simulink model "StraightACC_cs_old"  (R2016a)
settings: Solver=ode5  SolverMode=SingleTasking  StartTime=0.0  StopTime=10  FixedStep=1/1000  RelTol=1e-3
PreLoadFcn:
  | mbxruntime.callbacks.PreLoadFcn(bdroot);
PostLoadFcn:
  | mbxruntime.callbacks.PostLoadFcn(bdroot);
InitFcn:
  | mbxruntime.callbacks.InitFcn(bdroot);
StartFcn:
  | mbxruntime.callbacks.StartFcn(bdroot);
StopFcn:
  | mbxruntime.callbacks.StopFcn(bdroot);
model workspace (MAT data in the model file):
  mbox_table : struct (value not decoded)
  model_closed = 0
  sim_status = 0
values from neighbouring files (symbols this model uses):
  CCCDuration = 5    [PreScan_Runscript.m]
  V0 = CCCArray(2*CCCCasei-1)    [PreScan_Runscript.m]
  V1 = CCCArray(2*CCCCasei)    [PreScan_Runscript.m]
  VAccuracyIn = 0.8    [PreScan_Runscript.m]
  VDurationIn = 2    [PreScan_Runscript.m]
  VPIDIn = CCCArray(2*CCCCasei-1)    [PreScan_Runscript.m]
  VToleranceIn = 1    [PreScan_Runscript.m]
undefined symbols (not defined in the file or in its folder): ADASID, BMotor1, BMotor2, BrkDelayTime, DControlB, Delay1, Delay2, DiscIntNeverNeededParam, IControlB, JMotor1, JMotor2, PControlB, PreScanCarSimLoadFcn, ratioGearF, ratioGearR, TorqDelayTime, Tstep
undefined symbols (not defined in the file): WheelL0, WheelL1, WheelR0, WheelR1
libraries: simulink x13, simulink_extras x11, PreScanSimulinkLibrary x9, MyLib x3, Solver_SF x2, pil_lib x1, PreScanUsefulBlocks x1
(part 2 of 9)

== system StraightACC_cs_old/WheelL1_Roewe_550_S_Sedan_1 ==
  WheelL1_Roewe_550_S_Sedan_1 : Inport  Tag=inport/JointActuator  OutDataTypeStr=Bus: PRESCAN_POSE_DATA  SampleTime=10/1000  BusOutputAsStruct=on
  Actuator : Subsystem  Tag=VisuJoint  mask(PreScan Sink Block: VisuJoint){UniqueID=29, Translate_ObjectID3D=Roewe_550_S_Sedan_1.WheelL1, Rotate_ObjectID3D=Roewe_550_S_Sedan_1.WheelL1, TimeStep=10/1000, DisplayName=[]}
      mask prompts: UniqueID "Parent Unique ID"; Translate_ObjectID3D "Translate Object Name"; Rotate_ObjectID3D "Rotate Object Name"; TimeStep "Simulation Step"; DisplayName "Display Name"
      mask help:
      | The VisuJoint block provides a way to adapt the location and orientation of a part of an object.
      |
      | For more information, please click Help.
      settings: DeleteFcn=PreScanBlockDeleteFcn;
      mask Help: eval('openHelp(223)')
      mask Display: image(imread('Joint.png'))
  wires:
  WheelL1_Roewe_550_S_Sedan_1/1 -> Actuator/1(Joint)

== system StraightACC_cs_old/WheelR0_Roewe_550_S_Sedan_1 ==
  WheelR0_Roewe_550_S_Sedan_1 : Inport  Tag=inport/JointActuator  OutDataTypeStr=Bus: PRESCAN_POSE_DATA  SampleTime=10/1000  BusOutputAsStruct=on
  Actuator : Subsystem  Tag=VisuJoint  mask(PreScan Sink Block: VisuJoint){UniqueID=29, Translate_ObjectID3D=Roewe_550_S_Sedan_1.WheelR0, Rotate_ObjectID3D=Roewe_550_S_Sedan_1.WheelR0, TimeStep=10/1000, DisplayName=[]}
      mask prompts: UniqueID "Parent Unique ID"; Translate_ObjectID3D "Translate Object Name"; Rotate_ObjectID3D "Rotate Object Name"; TimeStep "Simulation Step"; DisplayName "Display Name"
      mask help:
      | The VisuJoint block provides a way to adapt the location and orientation of a part of an object.
      |
      | For more information, please click Help.
      settings: DeleteFcn=PreScanBlockDeleteFcn;
      mask Help: eval('openHelp(223)')
      mask Display: image(imread('Joint.png'))
  wires:
  WheelR0_Roewe_550_S_Sedan_1/1 -> Actuator/1(Joint)

== system StraightACC_cs_old/WheelR1_Roewe_550_S_Sedan_1 ==
  WheelR1_Roewe_550_S_Sedan_1 : Inport  Tag=inport/JointActuator  OutDataTypeStr=Bus: PRESCAN_POSE_DATA  SampleTime=10/1000  BusOutputAsStruct=on
  Actuator : Subsystem  Tag=VisuJoint  mask(PreScan Sink Block: VisuJoint){UniqueID=29, Translate_ObjectID3D=Roewe_550_S_Sedan_1.WheelR1, Rotate_ObjectID3D=Roewe_550_S_Sedan_1.WheelR1, TimeStep=10/1000, DisplayName=[]}
      mask prompts: UniqueID "Parent Unique ID"; Translate_ObjectID3D "Translate Object Name"; Rotate_ObjectID3D "Rotate Object Name"; TimeStep "Simulation Step"; DisplayName "Display Name"
      mask help:
      | The VisuJoint block provides a way to adapt the location and orientation of a part of an object.
      |
      | For more information, please click Help.
      settings: DeleteFcn=PreScanBlockDeleteFcn;
      mask Help: eval('openHelp(223)')
      mask Display: image(imread('Joint.png'))
  wires:
  WheelR1_Roewe_550_S_Sedan_1/1 -> Actuator/1(Joint)

== system StraightACC_cs_old/Audi_A8_Sedan_1/SELF_Demux ==
  SELF : Inport  OutDataTypeStr=Bus: PRESCAN_SELFSENSORDATA
  Bus Selector : BusSelector  OutputSignals=PositionX,PositionY,PositionZ,OrientationRoll,OrientationPitch,OrientationYaw,Velocity,Yaw_rate,Lat,Long,Alt
  Demux2 : Demux  Outputs=3
  Gain : Gain  Gain=180/pi
  Gain1 : Gain  Gain=180/pi
  Vector Concatenate1 : Concatenate  NumInputs=3
  compas converter : Subsystem
  x [m] : Outport
  y [m] : Outport  Port=2
  z [m] : Outport  Port=3
  rotx [deg] : Outport  Port=4
  roty [deg] : Outport  Port=5
  rotz [deg] : Outport  Port=6
  GPS lat [deg] : Outport  Port=7
  GPS long [deg] : Outport  Port=8
  GPS alt [m] : Outport  Port=9
  velocity [m/s] : Outport  Port=10
  heading [deg] : Outport  Port=11
  yaw rate [deg/s] : Outport  Port=12
  wires:
  Bus Selector/11 -> GPS alt [m]/1  "<Alt>"
  Bus Selector/10 -> GPS long [deg]/1  "<Long>"
  Bus Selector/9 -> GPS lat [deg]/1  "<Lat>"
  Bus Selector/8 -> Gain1/1  "<Yaw_rate>"
  Bus Selector/7 -> velocity [m/s]/1  "<Velocity>"
  Bus Selector/6 -> compas converter/1(rotz [rad]), Vector Concatenate1/3  "<OrientationYaw>"
  Bus Selector/5 -> Vector Concatenate1/2  "<OrientationPitch>"
  Bus Selector/4 -> Vector Concatenate1/1  "<OrientationRoll>"
  Vector Concatenate1/1 -> Gain/1
  Bus Selector/3 -> z [m]/1  "<PositionZ>"
  Bus Selector/2 -> y [m]/1  "<PositionY>"
  Bus Selector/1 -> x [m]/1  "<PositionX>"
  SELF/1 -> Bus Selector/1
  Gain/1 -> Demux2/1
  Demux2/1 -> rotx [deg]/1
  Demux2/2 -> roty [deg]/1
  Demux2/3 -> rotz [deg]/1
  compas converter/1(heading [deg]) -> heading [deg]/1
  Gain1/1 -> yaw rate [deg/s]/1

== system StraightACC_cs_old/Audi_A8_Sedan_1/STATE_Audi_A8_Sedan_1 ==
  State : Inport  SampleTime=TimeStep
  Bus Creator : BusCreator  Inputs=15  OutDataTypeStr=Bus: PRESCAN_STATEACTUATORDATA  NonVirtualBus=on
  Demux : Demux  Outputs=15
  iniBODYAngles wrtVEH [rad] : Constant  Value=[Roll0 Pitch0 0]  SampleTime=TimeStep
  iniVEHAngles wrtGLOB [rad] : Constant  Value=[0 0 Yaw0]  SampleTime=TimeStep
  iniVEHposition wrtGLOB [m] : Constant  Value=[x0 y0 z0]  SampleTime=TimeStep
  state2FullState : PreScanSimulinkLibrary/state2FullState  SystemSampleTime=-1
  StateBus : Outport  OutDataTypeStr=Bus: PRESCAN_STATEACTUATORDATA
  wires:
  Bus Creator/1 -> StateBus/1
  State/1 -> state2FullState/1
  state2FullState/1 -> Demux/1
  iniVEHposition wrtGLOB [m]/1 -> state2FullState/2
  iniBODYAngles wrtVEH [rad]/1 -> state2FullState/3
  iniVEHAngles wrtGLOB [rad]/1 -> state2FullState/4
  Demux/1 -> Bus Creator/1  "PositionX"
  Demux/2 -> Bus Creator/2  "PositionY"
  Demux/3 -> Bus Creator/3  "PositionZ"
  Demux/4 -> Bus Creator/4  "VelocityX"
  Demux/5 -> Bus Creator/5  "VelocityY"
  Demux/6 -> Bus Creator/6  "VelocityZ"
  Demux/7 -> Bus Creator/7  "AccelerationX"
  Demux/8 -> Bus Creator/8  "AccelerationY"
  Demux/9 -> Bus Creator/9  "AccelerationZ"
  Demux/10 -> Bus Creator/10  "OrientationRoll"
  Demux/11 -> Bus Creator/11  "OrientationPitch"
  Demux/12 -> Bus Creator/12  "OrientationYaw"
  Demux/13 -> Bus Creator/13  "AngularVelocityRoll"
  Demux/14 -> Bus Creator/14  "AngularVelocityPitch"
  Demux/15 -> Bus Creator/15  "AngularVelocityYaw"

== system StraightACC_cs_old/Audi_A8_Sedan_1/Trajectories ==
  Traj2State1 : Subsystem  Tag=Traj2State  mask(PreScan Demux Block:){}
      settings: DeleteFcn=PreScanBlockDeleteFcn;
  TrajCoGOffset : Subsystem  Tag=TrajCoGOffset  mask(Trajectory CoG Offset block){CoGOffsetZ=0.55, InitRoll=0, InitPitch=0}
      mask prompts: CoGOffsetZ "Z-component of CoG Offset [m]:"; InitRoll "Initial Roll angle [deg]:"; InitPitch "Initial Pitch angle [deg]:"
      mask help: A trajectory follows the surface of the road. However the position of a actor is based on the actor's Center of Gravity, which is typically above the road. This block converts from the trajectory along the road surface to the trajectory of the actor's CoG by realigning the z-component of the CoG offset to be normal to the road.
      settings: DeleteFcn=PreScanBlockDeleteFcn;
  Trajectory_1 : Subsystem  Tag=Trajectory  mask(PreScan Source Block: Trajectory){FileName='Trajectory_1.mat', TimeStep=10/1000}
      mask prompts: TimeStep "Time Step [s]"
      mask help:
      | The Trajectory block contains the trajectories defined in the PreScan Experiment Editor. The output of the trajectory block is the (vehicle) State.
      |
      | For more information, please click Help.
      mask init:
      | EXPROOT=pwd;  % TODO better construction for locating base experiment
      | 
      | trajfilename = fullfile(EXPROOT,'Trajectories',FileName);
      | load(trajfilename);
      | trajectory=trajectory';
      | 
      | traj.time=trajectory(:,1);%[];
      | traj.signals.values=trajectory(:,2:19);
      | traj.dimensions=18;
      | traj.label='';
      | 
      | SampleTime=traj.time(2)-traj.time(1);
      settings: DeleteFcn=PreScanBlockDeleteFcn;
      mask Help: eval('openHelp(312)')
      mask Display: fprintf(FileName)
  Trajectory_1_Offset : Constant  Tag=TrajectoryOffset  Value="[0  0  0  0  0  0]"
  State : Outport  Tag=TrajOutport
  wires:
  Trajectory_1/1(trajectory) -> Traj2State1/1(Traj Org)
  Trajectory_1_Offset/1 -> Traj2State1/2(Offset)
  TrajCoGOffset/1(State Out) -> State/1
  Traj2State1/1(state) -> TrajCoGOffset/1(State In)

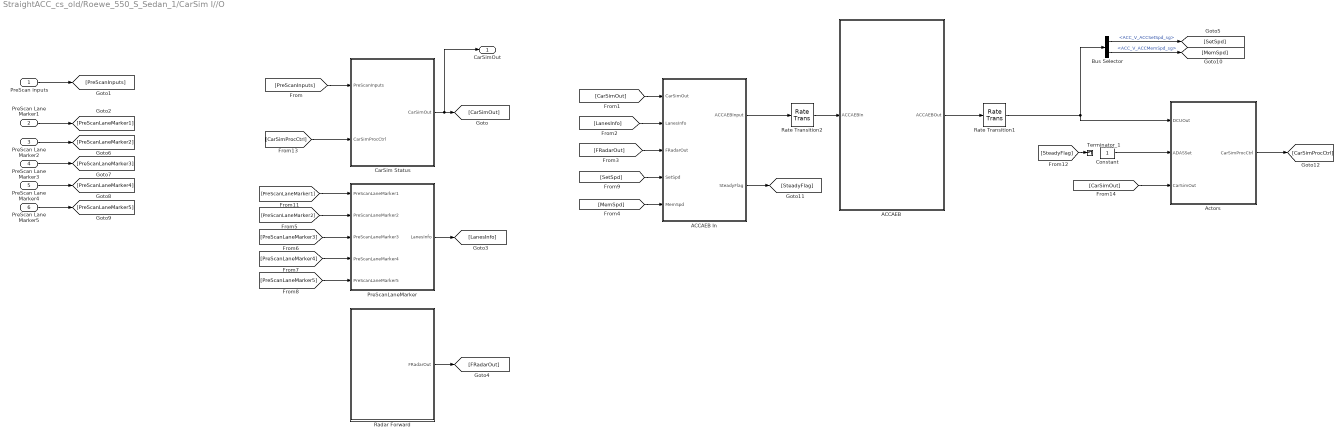
== system StraightACC_cs_old/Roewe_550_S_Sedan_1/CarSim I//O ==
  PreScan inputs : Inport
  PreScan Lane Marker1 : Inport  Port=2
  PreScan Lane Marker2 : Inport  Port=3
  PreScan Lane Marker3 : Inport  Port=4
  PreScan Lane Marker4 : Inport  Port=5
  PreScan Lane Marker5 : Inport  Port=6
  ACCAEB : Subsystem  DialogController=pil_create_dialog  LoadFcn=|
      | try
      |    if ~strcmp(rtw.pil.getPILVersion, '6.10 (R2016a)_12')
      |       set_param(gcb, 'DialogController', '');
      |       set_param(gcb, 'DialogControllerArgs', '');
      |    end
      | catch e
      |       set_param(gcb, 'DialogController', '');
      |       set_param(gcb, 'DialogControllerArgs', '');
      | end
      mask help: PIL:pil:XILBlockMaskDesc
      mask Display: disp('SIL S-Function');
  ACCAEB In : Subsystem  TreatAsAtomicUnit=on
  Actors : Subsystem
  Bus Selector : BusSelector  OutputSignals=ACC_V_ACCSetSpd_sg,ACC_V_ACCMemSpd_sg
  "CarSim Status " : Subsystem  TreatAsAtomicUnit=on
  Constant : Constant
  PreScanLaneMarker : Subsystem  TreatAsAtomicUnit=on
  Radar Forward : Subsystem  TreatAsAtomicUnit=on
  Rate Transition1 : RateTransition  OutPortSampleTime=0.001
  Rate Transition2 : RateTransition  OutPortSampleTime=0.01
  Terminator_1 : Terminator
  CarSimOut : Outport
  wires:
  [PreScanInputs] -> "CarSim Status "/1(PreScanInputs)
  PreScan inputs/1 -> [PreScanInputs]
  PreScan Lane Marker1/1 -> [PreScanLaneMarker1]
  "CarSim Status "/1(CarSimOut) -> CarSimOut/1, [CarSimOut]
  [PreScanLaneMarker1] -> PreScanLaneMarker/1(PreScanLaneMarker1)
  [CarSimOut] -> ACCAEB In/1(CarSimOut)
  PreScanLaneMarker/1(LanesInfo) -> [LanesInfo]
  [LanesInfo] -> ACCAEB In/2(LanesInfo)
  Radar Forward/1(FRadarOut) -> [FRadarOut]
  [FRadarOut] -> ACCAEB In/3(FRadarOut)
  [CarSimProcCtrl] -> "CarSim Status "/2(CarSimProcCtrl)
  PreScan Lane Marker2/1 -> [PreScanLaneMarker2]
  PreScan Lane Marker3/1 -> [PreScanLaneMarker3]
  PreScan Lane Marker4/1 -> [PreScanLaneMarker4]
  PreScan Lane Marker5/1 -> [PreScanLaneMarker5]
  [PreScanLaneMarker2] -> PreScanLaneMarker/2(PreScanLaneMarker2)
  [PreScanLaneMarker3] -> PreScanLaneMarker/3(PreScanLaneMarker3)
  [PreScanLaneMarker4] -> PreScanLaneMarker/4(PreScanLaneMarker4)
  [PreScanLaneMarker5] -> PreScanLaneMarker/5(PreScanLaneMarker5)
  Rate Transition2/1 -> ACCAEB/1(ACCAEBIn)
  ACCAEB In/1(ACCAEBInput) -> Rate Transition2/1
  ACCAEB/1(ACCAEBOut) -> Rate Transition1/1
  Rate Transition1/1 -> Bus Selector/1, Actors/1(DCUOut)
  ACCAEB In/2(SteadyFlag) -> [SteadyFlag]
  [CarSimOut] -> Actors/3(CarSimOut)
  Actors/1(CarSimProcCtrl) -> [CarSimProcCtrl]
  Constant/1 -> Actors/2(ADASSet)
  Bus Selector/1 -> [SetSpd]  "<ACC_V_ACCSetSpd_sg>"
  Bus Selector/2 -> [MemSpd]  "<ACC_V_ACCMemSpd_sg>"
  [SetSpd] -> ACCAEB In/4(SetSpd)
  [MemSpd] -> ACCAEB In/5(MemSpd)
  [SteadyFlag] -> Terminator_1/1

== system StraightACC_cs_old/Roewe_550_S_Sedan_1/CarSim_Vehicle ==
  note: For state mode 'Dynamic' positions
      | are not taken into account, as they
      | are computed by integrating velocity.
      | Click annotation for Help.
  Contact_In : Inport
  CarSim S-Function2 : Solver_SF/CarSim S-Function2  Priority=1  VehicleCode=i_i  SIMFILE=simfile.sim
      settings: AttributesFormatString=Vehicle Code: %<VehicleCode>
  CarSim2PreScanSTATE : Subsystem  Tag=CarSim2PreScanSTATE  mask(CarSim2PreScan:){z0=0}
      mask prompts: z0 "PreScan Actor initial COG z-position wrt GLOBAL axis system [m]"
      mask help: This block converts the outputs coming from the CarSim block into consistent PreScan signals.
  CarSim2PreScan_BUS : Subsystem  Tag=CarSim2PreScan_BUS  mask(PreScan block: CarSim to PreScan BUS){TyreRadius=0.44999998807907104, cogZOffset=0}
      mask prompts: TyreRadius "Tyre Radius [m]"; cogZOffset "cog Z offset [m]"
      mask help: CarSim to PreScan BUS selector
      mask Help: eval('openHelp()')
      mask Display: disp('PreScan BUS\nVehicleDynamics')
  CarSim2PreScan_ContactAdapter : Subsystem  Tag=CarSim2PreScan_ContactAdapter  mask{wheelRadius=0.44999998807907104}
      mask prompts: wheelRadius "Wheel radius:"
  MuxState : Subsystem  Tag=mux/State  mask(Empty Dynamics State Block){positioningmode=on, TimeStep=1/1000}
      mask prompts: positioningmode "Positioning Mode"; TimeStep "Auto Assigned: Time Step [s]"
      mask help:
      | Build the state of an actor based on user input.
      | The user can either use positioning mode or dynamics mode.
      | - When using positioning mode the position and orientation of the actor are set directly based on the input. Expected input is relative to the initial position and orientation of the actor. It's also possible to specify the velocity of the actor, though this input isn't used, only passed on.
      | - When using dynamics mode the position input is ignored. Expected input is velocity and orientation. The velocity is relative the current orientation of the actor, while orientation is relative to its initial orientation. The position of the actor is calculated based on the velocity and orientation given.
      settings: DeleteFcn=PreScanBlockDeleteFcn;
  TyreContact To Road Information : Subsystem  Tag=TyreContactToRoadInformation  mask{Roll0=0, Pitch0=0, Yaw0=0}
      mask prompts: Roll0 "Ini roll-angle BODY wrt VEHICLE axis system [deg]"; Pitch0 "Ini pitch-angle BODY wrt VEHICLE axis system [deg]"; Yaw0 "Ini yaw-angle VEHICLE wrt GLOBAL axis system [deg]"
  State : Outport
  State_BUS : Outport  Port=2
  ContactParams : Outport  Port=3
  wires:
  MuxState/1(state) -> State/1, CarSim2PreScan_ContactAdapter/1(State)
  CarSim2PreScanSTATE/1(x [m]) -> MuxState/1(x [m])
  CarSim2PreScanSTATE/2(y [m]) -> MuxState/2(y [m])
  CarSim2PreScanSTATE/3(z [m]) -> MuxState/3(z [m])
  CarSim2PreScanSTATE/4(dx [m/s]) -> MuxState/4(dx [m/s])
  CarSim2PreScanSTATE/5(dy [m/s]) -> MuxState/5(dy [m/s])
  CarSim2PreScanSTATE/6(dz [m/s]) -> MuxState/6(dz [m/s])
  CarSim2PreScanSTATE/7(R [rad]) -> MuxState/7(R [rad])
  CarSim2PreScanSTATE/8(P [rad]) -> MuxState/8(P [rad])
  CarSim2PreScanSTATE/9(Y [rad]) -> MuxState/9(Y [rad])
  CarSim2PreScan_BUS/1(PreScanBUS_VehicleDynamics) -> State_BUS/1, CarSim2PreScan_ContactAdapter/2(State_Bus)
  CarSim S-Function2/1 -> CarSim2PreScanSTATE/1(CarSim_In), CarSim2PreScan_BUS/1(CarSim_In)
  Contact_In/1 -> TyreContact To Road Information/1(TyreInfo_in)
  CarSim2PreScan_ContactAdapter/1(ContactParams) -> ContactParams/1

== system StraightACC_cs_old/Roewe_550_S_Sedan_1/LaneMarkerSensor_1_Data ==
  In1 : Inport
  Bus Creator : BusCreator  Inputs='SliceCount','ScanAtSensor','ScanAtDistance1','ScanAtDistance2','ScanAtDistance3'
  Constant : Constant
  Constant1 : Constant  Value=NUMBEROFSLICES
  Constant2 : Constant  Value=2
  Constant3 : Constant  Value=3
  Constant4 : Constant  Value=4
  Data Type Conversion : DataTypeConversion  OutDataTypeStr=int32
  If{,1..3} (4 alike) : If  NumInputs=2  IfExpression=u1 >= u2  ShowElse=off
  If Action Subsystem1 : Subsystem  TreatAsAtomicUnit=on
  If Action Subsystem2 : Subsystem  TreatAsAtomicUnit=on
  If Action Subsystem3 : Subsystem  TreatAsAtomicUnit=on
  If Action Subsystem4 : Subsystem  TreatAsAtomicUnit=on
  Merge{,1..3} (4 alike) : Merge  InitialOutput=0
  Zero-filled data bus{,1..3} (4 alike) : Constant  Value=0  VectorParams1D=off  OutDataTypeStr=Bus: PRESCAN_LANEMARKER_DATA  SampleTime=TimeStep
  Detection Data : Outport
  wires:
  Data Type Conversion/1 -> Bus Creator/1  "SliceCount"
  In1/1 -> If Action Subsystem2/1(In1), If Action Subsystem4/1(In1), If Action Subsystem3/1(In1), If Action Subsystem1/1(In1)
  Zero-filled data bus3/1 -> Merge3/1
  Zero-filled data bus2/1 -> Merge2/1
  Zero-filled data bus1/1 -> Merge1/1
  Zero-filled data bus/1 -> Merge/1
  Merge3/1 -> Bus Creator/5  "ScanAtDistance3"
  Merge2/1 -> Bus Creator/4  "ScanAtDistance2"
  Merge1/1 -> Bus Creator/3  "ScanAtDistance1"
  If3/1 -> If Action Subsystem4/Action
  If Action Subsystem4/1(Out1) -> Merge3/2
  Constant4/1 -> If3/2, If Action Subsystem4/2(In2)
  If2/1 -> If Action Subsystem3/Action
  If Action Subsystem3/1(Out1) -> Merge2/2
  Constant3/1 -> If Action Subsystem3/2(In2), If2/2
  If1/1 -> If Action Subsystem1/Action
  If Action Subsystem1/1(Out1) -> Merge1/2
  Constant2/1 -> If Action Subsystem1/2(In2), If1/2
  Merge/1 -> Bus Creator/2  "ScanAtSensor"
  Bus Creator/1 -> Detection Data/1
  If/1 -> If Action Subsystem2/Action
  If Action Subsystem2/1(Out1) -> Merge/2
  Constant/1 -> If Action Subsystem2/2(In2), If/2
  Constant1/1 -> Data Type Conversion/1, If3/1, If2/1, If1/1, If/1

== system StraightACC_cs_old/Roewe_550_S_Sedan_1/LaneMarkerSensor_2_Data ==
  In1 : Inport
  Bus Creator : BusCreator  Inputs='SliceCount','ScanAtSensor','ScanAtDistance1','ScanAtDistance2','ScanAtDistance3'
  Constant : Constant
  Constant1 : Constant  Value=NUMBEROFSLICES
  Constant2 : Constant  Value=2
  Constant3 : Constant  Value=3
  Constant4 : Constant  Value=4
  Data Type Conversion : DataTypeConversion  OutDataTypeStr=int32
  If{,1..3} (4 alike) : If  NumInputs=2  IfExpression=u1 >= u2  ShowElse=off
  If Action Subsystem1 : Subsystem  TreatAsAtomicUnit=on
  If Action Subsystem2 : Subsystem  TreatAsAtomicUnit=on
  If Action Subsystem3 : Subsystem  TreatAsAtomicUnit=on
  If Action Subsystem4 : Subsystem  TreatAsAtomicUnit=on
  Merge{,1..3} (4 alike) : Merge  InitialOutput=0
  Zero-filled data bus{,1..3} (4 alike) : Constant  Value=0  VectorParams1D=off  OutDataTypeStr=Bus: PRESCAN_LANEMARKER_DATA  SampleTime=TimeStep
  Detection Data : Outport
  wires:
  Data Type Conversion/1 -> Bus Creator/1  "SliceCount"
  In1/1 -> If Action Subsystem2/1(In1), If Action Subsystem4/1(In1), If Action Subsystem3/1(In1), If Action Subsystem1/1(In1)
  Zero-filled data bus3/1 -> Merge3/1
  Zero-filled data bus2/1 -> Merge2/1
  Zero-filled data bus1/1 -> Merge1/1
  Zero-filled data bus/1 -> Merge/1
  Merge3/1 -> Bus Creator/5  "ScanAtDistance3"
  Merge2/1 -> Bus Creator/4  "ScanAtDistance2"
  Merge1/1 -> Bus Creator/3  "ScanAtDistance1"
  If3/1 -> If Action Subsystem4/Action
  If Action Subsystem4/1(Out1) -> Merge3/2
  Constant4/1 -> If3/2, If Action Subsystem4/2(In2)
  If2/1 -> If Action Subsystem3/Action
  If Action Subsystem3/1(Out1) -> Merge2/2
  Constant3/1 -> If Action Subsystem3/2(In2), If2/2
  If1/1 -> If Action Subsystem1/Action
  If Action Subsystem1/1(Out1) -> Merge1/2
  Constant2/1 -> If Action Subsystem1/2(In2), If1/2
  Merge/1 -> Bus Creator/2  "ScanAtSensor"
  Bus Creator/1 -> Detection Data/1
  If/1 -> If Action Subsystem2/Action
  If Action Subsystem2/1(Out1) -> Merge/2
  Constant/1 -> If Action Subsystem2/2(In2), If/2
  Constant1/1 -> Data Type Conversion/1, If3/1, If2/1, If1/1, If/1

== system StraightACC_cs_old/Roewe_550_S_Sedan_1/LaneMarkerSensor_3_Data ==
  In1 : Inport
  Bus Creator : BusCreator  Inputs='SliceCount','ScanAtSensor','ScanAtDistance1','ScanAtDistance2','ScanAtDistance3'
  Constant : Constant
  Constant1 : Constant  Value=NUMBEROFSLICES
  Constant2 : Constant  Value=2
  Constant3 : Constant  Value=3
  Constant4 : Constant  Value=4
  Data Type Conversion : DataTypeConversion  OutDataTypeStr=int32
  If{,1..3} (4 alike) : If  NumInputs=2  IfExpression=u1 >= u2  ShowElse=off
  If Action Subsystem1 : Subsystem  TreatAsAtomicUnit=on
  If Action Subsystem2 : Subsystem  TreatAsAtomicUnit=on
  If Action Subsystem3 : Subsystem  TreatAsAtomicUnit=on
  If Action Subsystem4 : Subsystem  TreatAsAtomicUnit=on
  Merge{,1..3} (4 alike) : Merge  InitialOutput=0
  Zero-filled data bus{,1..3} (4 alike) : Constant  Value=0  VectorParams1D=off  OutDataTypeStr=Bus: PRESCAN_LANEMARKER_DATA  SampleTime=TimeStep
  Detection Data : Outport
  wires:
  Data Type Conversion/1 -> Bus Creator/1  "SliceCount"
  In1/1 -> If Action Subsystem2/1(In1), If Action Subsystem4/1(In1), If Action Subsystem3/1(In1), If Action Subsystem1/1(In1)
  Zero-filled data bus3/1 -> Merge3/1
  Zero-filled data bus2/1 -> Merge2/1
  Zero-filled data bus1/1 -> Merge1/1
  Zero-filled data bus/1 -> Merge/1
  Merge3/1 -> Bus Creator/5  "ScanAtDistance3"
  Merge2/1 -> Bus Creator/4  "ScanAtDistance2"
  Merge1/1 -> Bus Creator/3  "ScanAtDistance1"
  If3/1 -> If Action Subsystem4/Action
  If Action Subsystem4/1(Out1) -> Merge3/2
  Constant4/1 -> If3/2, If Action Subsystem4/2(In2)
  If2/1 -> If Action Subsystem3/Action
  If Action Subsystem3/1(Out1) -> Merge2/2
  Constant3/1 -> If Action Subsystem3/2(In2), If2/2
  If1/1 -> If Action Subsystem1/Action
  If Action Subsystem1/1(Out1) -> Merge1/2
  Constant2/1 -> If Action Subsystem1/2(In2), If1/2
  Merge/1 -> Bus Creator/2  "ScanAtSensor"
  Bus Creator/1 -> Detection Data/1
  If/1 -> If Action Subsystem2/Action
  If Action Subsystem2/1(Out1) -> Merge/2
  Constant/1 -> If Action Subsystem2/2(In2), If/2
  Constant1/1 -> Data Type Conversion/1, If3/1, If2/1, If1/1, If/1

== system StraightACC_cs_old/Roewe_550_S_Sedan_1/LaneMarkerSensor_4_Data ==
  In1 : Inport
  Bus Creator : BusCreator  Inputs='SliceCount','ScanAtSensor','ScanAtDistance1','ScanAtDistance2','ScanAtDistance3'
  Constant : Constant
  Constant1 : Constant  Value=NUMBEROFSLICES
  Constant2 : Constant  Value=2
  Constant3 : Constant  Value=3
  Constant4 : Constant  Value=4
  Data Type Conversion : DataTypeConversion  OutDataTypeStr=int32
  If{,1..3} (4 alike) : If  NumInputs=2  IfExpression=u1 >= u2  ShowElse=off
  If Action Subsystem1 : Subsystem  TreatAsAtomicUnit=on
  If Action Subsystem2 : Subsystem  TreatAsAtomicUnit=on
  If Action Subsystem3 : Subsystem  TreatAsAtomicUnit=on
  If Action Subsystem4 : Subsystem  TreatAsAtomicUnit=on
  Merge{,1..3} (4 alike) : Merge  InitialOutput=0
  Zero-filled data bus{,1..3} (4 alike) : Constant  Value=0  VectorParams1D=off  OutDataTypeStr=Bus: PRESCAN_LANEMARKER_DATA  SampleTime=TimeStep
  Detection Data : Outport
  wires:
  Data Type Conversion/1 -> Bus Creator/1  "SliceCount"
  In1/1 -> If Action Subsystem2/1(In1), If Action Subsystem4/1(In1), If Action Subsystem3/1(In1), If Action Subsystem1/1(In1)
  Zero-filled data bus3/1 -> Merge3/1
  Zero-filled data bus2/1 -> Merge2/1
  Zero-filled data bus1/1 -> Merge1/1
  Zero-filled data bus/1 -> Merge/1
  Merge3/1 -> Bus Creator/5  "ScanAtDistance3"
  Merge2/1 -> Bus Creator/4  "ScanAtDistance2"
  Merge1/1 -> Bus Creator/3  "ScanAtDistance1"
  If3/1 -> If Action Subsystem4/Action
  If Action Subsystem4/1(Out1) -> Merge3/2
  Constant4/1 -> If3/2, If Action Subsystem4/2(In2)
  If2/1 -> If Action Subsystem3/Action
  If Action Subsystem3/1(Out1) -> Merge2/2
  Constant3/1 -> If Action Subsystem3/2(In2), If2/2
  If1/1 -> If Action Subsystem1/Action
  If Action Subsystem1/1(Out1) -> Merge1/2
  Constant2/1 -> If Action Subsystem1/2(In2), If1/2
  Merge/1 -> Bus Creator/2  "ScanAtSensor"
  Bus Creator/1 -> Detection Data/1
  If/1 -> If Action Subsystem2/Action
  If Action Subsystem2/1(Out1) -> Merge/2
  Constant/1 -> If Action Subsystem2/2(In2), If/2
  Constant1/1 -> Data Type Conversion/1, If3/1, If2/1, If1/1, If/1

== system StraightACC_cs_old/Roewe_550_S_Sedan_1/LaneMarkerSensor_5_Data ==
  In1 : Inport
  Bus Creator : BusCreator  Inputs='SliceCount','ScanAtSensor','ScanAtDistance1','ScanAtDistance2','ScanAtDistance3'
  Constant : Constant
  Constant1 : Constant  Value=NUMBEROFSLICES
  Constant2 : Constant  Value=2
  Constant3 : Constant  Value=3
  Constant4 : Constant  Value=4
  Data Type Conversion : DataTypeConversion  OutDataTypeStr=int32
  If{,1..3} (4 alike) : If  NumInputs=2  IfExpression=u1 >= u2  ShowElse=off
  If Action Subsystem1 : Subsystem  TreatAsAtomicUnit=on
  If Action Subsystem2 : Subsystem  TreatAsAtomicUnit=on
  If Action Subsystem3 : Subsystem  TreatAsAtomicUnit=on
  If Action Subsystem4 : Subsystem  TreatAsAtomicUnit=on
  Merge{,1..3} (4 alike) : Merge  InitialOutput=0
  Zero-filled data bus{,1..3} (4 alike) : Constant  Value=0  VectorParams1D=off  OutDataTypeStr=Bus: PRESCAN_LANEMARKER_DATA  SampleTime=TimeStep
  Detection Data : Outport
  wires:
  Data Type Conversion/1 -> Bus Creator/1  "SliceCount"
  In1/1 -> If Action Subsystem2/1(In1), If Action Subsystem4/1(In1), If Action Subsystem3/1(In1), If Action Subsystem1/1(In1)
  Zero-filled data bus3/1 -> Merge3/1
  Zero-filled data bus2/1 -> Merge2/1
  Zero-filled data bus1/1 -> Merge1/1
  Zero-filled data bus/1 -> Merge/1
  Merge3/1 -> Bus Creator/5  "ScanAtDistance3"
  Merge2/1 -> Bus Creator/4  "ScanAtDistance2"
  Merge1/1 -> Bus Creator/3  "ScanAtDistance1"
  If3/1 -> If Action Subsystem4/Action
  If Action Subsystem4/1(Out1) -> Merge3/2
  Constant4/1 -> If3/2, If Action Subsystem4/2(In2)
  If2/1 -> If Action Subsystem3/Action
  If Action Subsystem3/1(Out1) -> Merge2/2
  Constant3/1 -> If Action Subsystem3/2(In2), If2/2
  If1/1 -> If Action Subsystem1/Action
  If Action Subsystem1/1(Out1) -> Merge1/2
  Constant2/1 -> If Action Subsystem1/2(In2), If1/2
  Merge/1 -> Bus Creator/2  "ScanAtSensor"
  Bus Creator/1 -> Detection Data/1
  If/1 -> If Action Subsystem2/Action
  If Action Subsystem2/1(Out1) -> Merge/2
  Constant/1 -> If Action Subsystem2/2(In2), If/2
  Constant1/1 -> Data Type Conversion/1, If3/1, If2/1, If1/1, If/1

== system StraightACC_cs_old/Roewe_550_S_Sedan_1/PreScan_RayCast_Contact_Sensor ==
  ContactParams : Inport  SampleTime=TimeStep
  Bus Creator2 : BusCreator  Inputs=4
  Constant : Constant  Value=0
  Contact Point Bus Creator : Subsystem
  Contact Point Bus Creator1 : Subsystem
  Contact Point Bus Creator2 : Subsystem
  Contact Point Bus Creator3 : Subsystem
  Demux : Demux
  Demux1 : Demux  Outputs=[9 1 12 4]
  Demux2 : Demux
  For All Wheel Contacts : Subsystem  TreatAsAtomicUnit=on
  Mux6 : Mux  Inputs=2
  Rate Transition : RateTransition  OutPortSampleTimeOpt=Inherit
  Subsystem1 : Subsystem  mask{NumberOfWheels=4, MaxContactPoints=1, Range=4}
      mask prompts: NumberOfWheels "Number of Wheels"; MaxContactPoints "Maximum number of Contact Points"
      mask Display: disp('RayCast Contact Sensor')
  Subsystem2 : Subsystem  mask{nrOfWheels=4}
      mask prompts: nrOfWheels "Number of Wheels:"
      mask Display:
      | port_label('input', 1,'Wheel poses')
      | port_label('input', 2,'Wheel radius')
      | port_label('input', 3,'Vehicle orientation')
      | 
      | port_label('output', 1,'Virtual poses')
  Vehicle Local to World : Subsystem
  Wheels = 4 : Subsystem  mask{NumberOfWheels=4}
      mask prompts: NumberOfWheels "Number of Wheels"
      mask Display:
      | port_label('input', 1,'Vehicle wrt World')
      | port_label('input', 2,'Wheels wrt World')
  Wheels Local to World : Subsystem  Tag=MuxWheels  mask(PreScan Mux Block:){}
      settings: DeleteFcn=PreScanBlockDeleteFcn;
  Results : Outport
  wires:
  Demux1/3 -> Demux2/1
  Demux1/1 -> Vehicle Local to World/1(State)
  ContactParams/1 -> Demux1/1
  Bus Creator2/1 -> Rate Transition/1
  Constant/1 -> Wheels Local to World/1(Steer Angle Front [deg]), Wheels Local to World/2(Steer Angle Rear [deg])
  Demux2/4 -> Wheels Local to World/7(Disp RR [m])
  Demux2/3 -> Wheels Local to World/6(Disp RL [m])
  Demux2/2 -> Wheels Local to World/5(Disp FR [m])
  Demux2/1 -> Wheels Local to World/4(Disp FL [m])
  Demux1/2 -> Wheels Local to World/3(Velocity [m/s])
  Wheels Local to World/1(Wheel Poses) -> Wheels = 4/2(Wheels wrt World)
  Vehicle Local to World/2(Orientation) -> Mux6/2, Subsystem2/3(Vehicle orientation)
  Vehicle Local to World/1(Position) -> Mux6/1
  Contact Point Bus Creator3/1(bus out) -> Bus Creator2/4  "TireRR"
  Contact Point Bus Creator2/1(bus out) -> Bus Creator2/3  "TireRL"
  Contact Point Bus Creator1/1(bus out) -> Bus Creator2/2  "TireFR"
  Contact Point Bus Creator/1(bus out) -> Bus Creator2/1  "TireFL"
  Demux/4 -> Contact Point Bus Creator3/1(demux in)
  Demux/3 -> Contact Point Bus Creator2/1(demux in)
  Demux/2 -> Contact Point Bus Creator1/1(demux in)
  Demux/1 -> Contact Point Bus Creator/1(demux in)
  Mux6/1 -> Wheels = 4/1(Vehicle wrt World)
  Rate Transition/1 -> Results/1
  Demux1/4 -> Subsystem2/2(Wheel radius)
  Wheels = 4/1(WheelPoses) -> Subsystem2/1(Wheel poses)
  Subsystem1/1(Out1) -> For All Wheel Contacts/1(In1)
  For All Wheel Contacts/1(Out1) -> Demux/1
  Subsystem2/1(Virtual Poses) -> Subsystem1/1(In1)

== system StraightACC_cs_old/Roewe_550_S_Sedan_1/PreScan_RayCast_Contact_Sensor1 ==
  ContactParams : Inport  SampleTime=TimeStep
  Bus Creator2 : BusCreator  Inputs=4
  Constant : Constant  Value=0
  Contact Point Bus Creator : Subsystem
  Contact Point Bus Creator1 : Subsystem
  Contact Point Bus Creator2 : Subsystem
  Contact Point Bus Creator3 : Subsystem
  Demux : Demux
  Demux1 : Demux  Outputs=[9 1 12 4]
  Demux2 : Demux
  For All Wheel Contacts : Subsystem  TreatAsAtomicUnit=on
  Mux6 : Mux  Inputs=2
  Rate Transition : RateTransition  OutPortSampleTimeOpt=Inherit
  Subsystem1 : Subsystem  mask{NumberOfWheels=4, MaxContactPoints=1, Range=4}
      mask prompts: NumberOfWheels "Number of Wheels"; MaxContactPoints "Maximum number of Contact Points"
      mask Display: disp('RayCast Contact Sensor')
  Subsystem2 : Subsystem  mask{nrOfWheels=4}
      mask prompts: nrOfWheels "Number of Wheels:"
      mask Display:
      | port_label('input', 1,'Wheel poses')
      | port_label('input', 2,'Wheel radius')
      | port_label('input', 3,'Vehicle orientation')
      | 
      | port_label('output', 1,'Virtual poses')
  Vehicle Local to World : Subsystem
  Wheels = 4 : Subsystem  mask{NumberOfWheels=4}
      mask prompts: NumberOfWheels "Number of Wheels"
      mask Display:
      | port_label('input', 1,'Vehicle wrt World')
      | port_label('input', 2,'Wheels wrt World')
  Wheels Local to World : Subsystem  Tag=MuxWheels  mask(PreScan Mux Block:){}
      settings: DeleteFcn=PreScanBlockDeleteFcn;
  Results : Outport
  wires:
  Demux1/3 -> Demux2/1
  Demux1/1 -> Vehicle Local to World/1(State)
  ContactParams/1 -> Demux1/1
  Bus Creator2/1 -> Rate Transition/1
  Constant/1 -> Wheels Local to World/1(Steer Angle Front [deg]), Wheels Local to World/2(Steer Angle Rear [deg])
  Demux2/4 -> Wheels Local to World/7(Disp RR [m])
  Demux2/3 -> Wheels Local to World/6(Disp RL [m])
  Demux2/2 -> Wheels Local to World/5(Disp FR [m])
  Demux2/1 -> Wheels Local to World/4(Disp FL [m])
  Demux1/2 -> Wheels Local to World/3(Velocity [m/s])
  Wheels Local to World/1(Wheel Poses) -> Wheels = 4/2(Wheels wrt World)
  Vehicle Local to World/2(Orientation) -> Mux6/2, Subsystem2/3(Vehicle orientation)
  Vehicle Local to World/1(Position) -> Mux6/1
  Contact Point Bus Creator3/1(bus out) -> Bus Creator2/4  "TireRR"
  Contact Point Bus Creator2/1(bus out) -> Bus Creator2/3  "TireRL"
  Contact Point Bus Creator1/1(bus out) -> Bus Creator2/2  "TireFR"
  Contact Point Bus Creator/1(bus out) -> Bus Creator2/1  "TireFL"
  Demux/4 -> Contact Point Bus Creator3/1(demux in)
  Demux/3 -> Contact Point Bus Creator2/1(demux in)
  Demux/2 -> Contact Point Bus Creator1/1(demux in)
  Demux/1 -> Contact Point Bus Creator/1(demux in)
  Mux6/1 -> Wheels = 4/1(Vehicle wrt World)
  Rate Transition/1 -> Results/1
  Demux1/4 -> Subsystem2/2(Wheel radius)
  Wheels = 4/1(WheelPoses) -> Subsystem2/1(Wheel poses)
  Subsystem1/1(Out1) -> For All Wheel Contacts/1(In1)
  For All Wheel Contacts/1(Out1) -> Demux/1
  Subsystem2/1(Virtual Poses) -> Subsystem1/1(In1)

== system StraightACC_cs_old/Roewe_550_S_Sedan_1/SELF_Demux ==
  SELF : Inport  OutDataTypeStr=Bus: PRESCAN_SELFSENSORDATA
  Bus Selector : BusSelector  OutputSignals=PositionX,PositionY,PositionZ,OrientationRoll,OrientationPitch,OrientationYaw,Velocity,Yaw_rate,Lat,Long,Alt
  Demux2 : Demux  Outputs=3
  Gain : Gain  Gain=180/pi
  Gain1 : Gain  Gain=180/pi
  Vector Concatenate1 : Concatenate  NumInputs=3
  compas converter : Subsystem
  x [m] : Outport
  y [m] : Outport  Port=2
  z [m] : Outport  Port=3
  rotx [deg] : Outport  Port=4
  roty [deg] : Outport  Port=5
  rotz [deg] : Outport  Port=6
  GPS lat [deg] : Outport  Port=7
  GPS long [deg] : Outport  Port=8
  GPS alt [m] : Outport  Port=9
  velocity [m/s] : Outport  Port=10
  heading [deg] : Outport  Port=11
  yaw rate [deg/s] : Outport  Port=12
  wires:
  Bus Selector/11 -> GPS alt [m]/1  "<Alt>"
  Bus Selector/10 -> GPS long [deg]/1  "<Long>"
  Bus Selector/9 -> GPS lat [deg]/1  "<Lat>"
  Bus Selector/8 -> Gain1/1  "<Yaw_rate>"
  Bus Selector/7 -> velocity [m/s]/1  "<Velocity>"
  Bus Selector/6 -> compas converter/1(rotz [rad]), Vector Concatenate1/3  "<OrientationYaw>"
  Bus Selector/5 -> Vector Concatenate1/2  "<OrientationPitch>"
  Bus Selector/4 -> Vector Concatenate1/1  "<OrientationRoll>"
  Vector Concatenate1/1 -> Gain/1
  Bus Selector/3 -> z [m]/1  "<PositionZ>"
  Bus Selector/2 -> y [m]/1  "<PositionY>"
  Bus Selector/1 -> x [m]/1  "<PositionX>"
  SELF/1 -> Bus Selector/1
  Gain/1 -> Demux2/1
  Demux2/1 -> rotx [deg]/1
  Demux2/2 -> roty [deg]/1
  Demux2/3 -> rotz [deg]/1
  compas converter/1(heading [deg]) -> heading [deg]/1
  Gain1/1 -> yaw rate [deg/s]/1

== system StraightACC_cs_old/Roewe_550_S_Sedan_1/STATE_Roewe_550_S_Sedan_1 ==
  State : Inport  SampleTime=TimeStep
  Bus Creator : BusCreator  Inputs=15  OutDataTypeStr=Bus: PRESCAN_STATEACTUATORDATA  NonVirtualBus=on
  Demux : Demux  Outputs=15
  iniBODYAngles wrtVEH [rad] : Constant  Value=[Roll0 Pitch0 0]  SampleTime=TimeStep
  iniVEHAngles wrtGLOB [rad] : Constant  Value=[0 0 Yaw0]  SampleTime=TimeStep
  iniVEHposition wrtGLOB [m] : Constant  Value=[x0 y0 z0]  SampleTime=TimeStep
  state2FullState : PreScanSimulinkLibrary/state2FullState  SystemSampleTime=-1
  StateBus : Outport  OutDataTypeStr=Bus: PRESCAN_STATEACTUATORDATA
  wires:
  Bus Creator/1 -> StateBus/1
  State/1 -> state2FullState/1
  state2FullState/1 -> Demux/1
  iniVEHposition wrtGLOB [m]/1 -> state2FullState/2
  iniBODYAngles wrtVEH [rad]/1 -> state2FullState/3
  iniVEHAngles wrtGLOB [rad]/1 -> state2FullState/4
  Demux/1 -> Bus Creator/1  "PositionX"
  Demux/2 -> Bus Creator/2  "PositionY"
  Demux/3 -> Bus Creator/3  "PositionZ"
  Demux/4 -> Bus Creator/4  "VelocityX"
  Demux/5 -> Bus Creator/5  "VelocityY"
  Demux/6 -> Bus Creator/6  "VelocityZ"
  Demux/7 -> Bus Creator/7  "AccelerationX"
  Demux/8 -> Bus Creator/8  "AccelerationY"
  Demux/9 -> Bus Creator/9  "AccelerationZ"
  Demux/10 -> Bus Creator/10  "OrientationRoll"
  Demux/11 -> Bus Creator/11  "OrientationPitch"
  Demux/12 -> Bus Creator/12  "OrientationYaw"
  Demux/13 -> Bus Creator/13  "AngularVelocityRoll"
  Demux/14 -> Bus Creator/14  "AngularVelocityPitch"
  Demux/15 -> Bus Creator/15  "AngularVelocityYaw"

== system StraightACC_cs_old/Roewe_550_S_Sedan_1/StateWheels2WheelDisplacementMuxCarSim ==
  StateWheels : Inport
  Average : Fcn  Expr=((u(1)+u(2))*0.5)*pi/180
  Average1 : Fcn  Expr=((u(1)+u(2))*0.5)*pi/180
  Average2 : Fcn  Expr=((u(1)+u(2))*0.5)*pi/180
  Bus Selector : BusSelector  OutputSignals=PreScanBUS_VehicleDynamics.Wheel.Position.Linear.Pos_FL_Wheel_CoorSys_V[x;y;z][m],PreScanBUS_VehicleDynamics.Wheel.Position.Angualr.Rot_FL_Wheel_CoorSys_V[x;y;z][deg].Angle_Camber_FL_Wheel_CoorSys_V[deg],PreScanBUS_VehicleDynamics.Wheel.Position.Angualr.Rot_FL_Wheel_CoorSys_V[x;y;z][deg].Angle_Rot_FL_Wheel[deg],PreScanBUS_VehicleDynamics.Wheel.Position.Angualr.Rot_FL_Wheel_CoorSys_V[x;y;z][deg].Angle_Toe_FL_Wheel_CoorSys_V[deg],PreScanBUS_VehicleDynamics.Wheel.Position.Linear.Pos_FR_Wheel_CoorSys_V[x;y;z][m],PreScanBUS_VehicleDynamics.Wheel.Position.Angualr.Rot_FR_Wheel_CoorSys_V[x;y;z][deg].Angle_Camber_FR_Wheel_CoorSys_V[deg],PreScanBUS_VehicleDynamics.Wheel.Position.Angualr.Rot_FR_Wheel_CoorSys_V[x;y;z][deg].Angle_Rot_FR_Wheel[deg],PreScanBUS_VehicleDynamics.Wheel.Position.Angualr.Rot_FR_Wheel_CoorSys_V[x;y;z][deg].Angle_Toe_FR_Wheel_CoorSys_V[deg],PreScanBUS_VehicleDynamics.Wheel.Position.Linear.Pos_RL_Wheel_CoorSys_V[x;y;z][m],PreScanBUS_VehicleDynamics.Wheel.Position.Angualr.Rot_RL_Wheel_CoorSys_V[x;y;z][deg].Angle_Camber_RL_Wheel_CoorSys_V[deg],PreScanBUS_VehicleDynamics.Wheel.Position.Angualr.Rot_RL_Wheel_CoorSys_V[x;y;z][deg].Angle_Rot_RL_Wheel[deg],PreScanBUS_VehicleDynamics.Wheel.Position.Angualr.Rot_RL_Wheel_CoorSys_V[x;y;z][deg].Angle_Toe_RL_Wheel_CoorSys_V[deg],PreScanBUS_VehicleDynamics.Wheel.Position.Linear.Pos_RR_Wheel_CoorSys_V[x;y;z][m],PreScanBUS_VehicleDynamics.Wheel.Position.Angualr.Rot_RR_Wheel_CoorSys_V[x;y;z][deg].Angle_Camber_RR_Wheel_CoorSys_V[deg],PreScanBUS_VehicleDynamics.Wheel.Position.Angualr.Rot_RR_Wheel_CoorSys_V[x;y;z][deg].Angle_Rot_RR_Wheel[deg],PreScanBUS_VehicleDynamics.Wheel.Position.Angualr.Rot_RR_Wheel_CoorSys_V[x;y;z][deg].Angle_Toe_RR_Wheel_CoorSys_V[deg]
  Demux{,1..3} (4 alike) : Demux  Outputs=3
  Mux : Mux  Inputs=2
  Mux1 : Mux  Inputs=2
  Mux2 : Mux  Inputs=2
  Terminator{,1..13} (14 alike) : Terminator
  Steering_Angle_Front_[rad] : Outport
  Steering_Angle_Rear_[rad] : Outport  Port=2
  WheelsRotation_[rad] : Outport  Port=3
  z displacement FL [m] : Outport  Port=4
  z displacement FR [m] : Outport  Port=5
  z displacement RL [m] : Outport  Port=6
  z displacement RR [m] : Outport  Port=7
  wires:
  Bus Selector/16 -> Mux1/2  "<Angle_Toe_RR_Wheel_CoorSys_V[deg]>"
  Bus Selector/12 -> Mux1/1  "<Angle_Toe_RL_Wheel_CoorSys_V[deg]>"
  Bus Selector/8 -> Mux/2  "<Angle_Toe_FR_Wheel_CoorSys_V[deg]>"
  Bus Selector/4 -> Mux/1  "<Angle_Toe_FL_Wheel_CoorSys_V[deg]>"
  Average2/1 -> WheelsRotation_[rad]/1
  Mux2/1 -> Average2/1
  Average1/1 -> Steering_Angle_Rear_[rad]/1
  Average/1 -> Steering_Angle_Front_[rad]/1
  Mux1/1 -> Average1/1
  Mux/1 -> Average/1
  Demux2/3 -> z displacement RL [m]/1  "z displacement RL [m]"
  Demux3/3 -> z displacement RR [m]/1  "z displacement RR [m]"
  Demux1/3 -> z displacement FR [m]/1  "z displacement FR [m]"
  Demux/3 -> z displacement FL [m]/1  "z displacement FL [m]"
  StateWheels/1 -> Bus Selector/1
  Bus Selector/1 -> Demux/1  "<Pos_FL_Wheel_CoorSys_V[x;y;z][m]>"
  Demux/1 -> Terminator/1
  Demux/2 -> Terminator1/1
  Bus Selector/2 -> Terminator8/1  "<Angle_Camber_FL_Wheel_CoorSys_V[deg]>"
  Bus Selector/3 -> Mux2/1  "<Angle_Rot_FL_Wheel[deg]>"
  Demux1/1 -> Terminator2/1
  Demux1/2 -> Terminator3/1
  Bus Selector/5 -> Demux1/1  "<Pos_FR_Wheel_CoorSys_V[x;y;z][m]>"
  Bus Selector/6 -> Terminator9/1  "<Angle_Camber_FR_Wheel_CoorSys_V[deg]>"
  Bus Selector/7 -> Mux2/2  "<Angle_Rot_FR_Wheel[deg]>"
  Demux2/1 -> Terminator4/1
  Demux2/2 -> Terminator5/1
  Bus Selector/9 -> Demux2/1  "<Pos_RL_Wheel_CoorSys_V[x;y;z][m]>"
  Bus Selector/10 -> Terminator10/1  "<Angle_Camber_RL_Wheel_CoorSys_V[deg]>"
  Bus Selector/11 -> Terminator11/1  "<Angle_Rot_RL_Wheel[deg]>"
  Demux3/1 -> Terminator6/1
  Demux3/2 -> Terminator7/1
  Bus Selector/13 -> Demux3/1  "<Pos_RR_Wheel_CoorSys_V[x;y;z][m]>"
  Bus Selector/14 -> Terminator12/1  "<Angle_Camber_RR_Wheel_CoorSys_V[deg]>"
  Bus Selector/15 -> Terminator13/1  "<Angle_Rot_RR_Wheel[deg]>"

== system StraightACC_cs_old/Roewe_550_S_Sedan_1/Subsystem ==
  Contact_In : Inport
  Constant : Constant  Value=ones(8,1)*0.85
  Mux : Mux  Inputs=[12 8]
  TyreContact To Road Information : Subsystem  Tag=TyreContactToRoadInformation  mask{Roll0=0, Pitch0=0, Yaw0=0}
      mask prompts: Roll0 "Ini roll-angle BODY wrt VEHICLE axis system [deg]"; Pitch0 "Ini pitch-angle BODY wrt VEHICLE axis system [deg]"; Yaw0 "Ini yaw-angle VEHICLE wrt GLOBAL axis system [deg]"
  PreScanInputs : Outport
  wires:
  Mux/1 -> PreScanInputs/1
  Constant/1 -> Mux/2
  TyreContact To Road Information/1(RoadSlopeAndZ_[FL;FR;RL;RR]) -> Mux/1
  Contact_In/1 -> TyreContact To Road Information/1(TyreInfo_in)

== system StraightACC_cs_old/Roewe_550_S_Sedan_1/Subsystem1 ==
  CarSimOut : Inport
  Bus Selector : BusSelector  OutputSignals=SprungMass_Pos_Global_x[m] (signal 1),SprungMass_Pos_Global_y[m] (signal 2),SprungMass_Pos_Global_z[m] (signal 3),VehicleCoG_Vx[km/h] (signal 4),VehicleCoG_Vy[km/h] (signal 5),VehicleCoG_Vz[km/h] (signal 6),SprungMass_Angle_Global_Roll[deg] (signal 7),SprungMass_Angle_Global_Pitch[deg] (signal 8),SprungMass_Angle_Global_Yaw[deg] (signal 9),CarSim_Pos_Wheel_FL_x[m] (signal 10),CarSim_Pos_Wheel_FL_y[m] (signal 11),CarSim_Pos_Wheel_FL_z[m] (signal 12),CarSim_Pos_Wheel_FR_x[m] (signal 13),CarSim_Pos_Wheel_FR_y[m] (signal 14),CarSim_Pos_Wheel_FR_z[m] (signal 15),CarSim_Pos_Wheel_RL_x[m] (signal 16),CarSim_Pos_Wheel_RL_y[m] (signal 17),CarSim_Pos_Wheel_RL_Z[m] (signal 18),CarSim_Pos_Wheel_RR_x[m] (signal 19),CarSim_Pos_Wheel_RR_y[m] (signal 20),CarSim_Pos_Wheel_RR_z[m] (signal 21),CarSim_Angle_Wheel_FL_Roll[deg] (signal 22),CarSim_Angle_Wheel_FL_Rot[rev] (signal 23),CarSim_Angle_Wheel_FL_Steer[deg] (signal 24),CarSim_Angle_Wheel_FR_Roll[deg] (signal 25),CarSim_Angle_Wheel_FR_Rot[rev] (signal 26),CarSim_Angle_Wheel_FR_Steer[deg] (signal 27),CarSim_Angle_Wheel_RL_Roll[deg] (signal 28),CarSim_Angle_Wheel_RL_Rot[rev] (signal 29),CarSim_Angle_Wheel_RL_Steer[deg] (signal 30),CarSim_Angle_Wheel_RR_Roll[deg] (signal 31),CarSim_Angle_Wheel_RR_Rot[rev] (signal 32),CarSim_Angle_Wheel_RR_Steer[deg] (signal 33),SteeringWheelAngle[deg] (signal 34),Axle1ReducedSW (signal 35)
  CarSim2PreScanSTATE : Subsystem  Tag=CarSim2PreScanSTATE  mask(CarSim2PreScan:){z0=0}
      mask prompts: z0 "PreScan Actor initial COG z-position wrt GLOBAL axis system [m]"
      mask help: This block converts the outputs coming from the CarSim block into consistent PreScan signals.
  CarSim2PreScan_BUS : Subsystem  Tag=CarSim2PreScan_BUS  mask(PreScan block: CarSim to PreScan BUS){TyreRadius=0.44999998807907104, cogZOffset=0}
      mask prompts: TyreRadius "Tyre Radius [m]"; cogZOffset "cog Z offset [m]"
      mask help: CarSim to PreScan BUS selector
      mask Help: eval('openHelp()')
      mask Display: disp('PreScan BUS\nVehicleDynamics')
  CarSim2PreScan_ContactAdapter : Subsystem  Tag=CarSim2PreScan_ContactAdapter  mask{wheelRadius=0.44999998807907104}
      mask prompts: wheelRadius "Wheel radius:"
  Demux : Demux  Outputs=[18 -1]
  Mux : Mux  Inputs=35
  MuxState : Subsystem  Tag=mux/State  mask(Empty Dynamics State Block){positioningmode=on, TimeStep=1/1000}
      mask prompts: positioningmode "Positioning Mode"; TimeStep "Auto Assigned: Time Step [s]"
      mask help:
      | Build the state of an actor based on user input.
      | The user can either use positioning mode or dynamics mode.
      | - When using positioning mode the position and orientation of the actor are set directly based on the input. Expected input is relative to the initial position and orientation of the actor. It's also possible to specify the velocity of the actor, though this input isn't used, only passed on.
      | - When using dynamics mode the position input is ignored. Expected input is velocity and orientation. The velocity is relative the current orientation of the actor, while orientation is relative to its initial orientation. The position of the actor is calculated based on the velocity and orientation given.
      settings: DeleteFcn=PreScanBlockDeleteFcn;
  Terminator_1 : Terminator
  State : Outport
  State_BUS : Outport  Port=2
  ContactParams : Outport  Port=3
  wires:
  MuxState/1(state) -> State/1, CarSim2PreScan_ContactAdapter/1(State)
  CarSim2PreScanSTATE/1(x [m]) -> MuxState/1(x [m])
  CarSim2PreScanSTATE/2(y [m]) -> MuxState/2(y [m])
  CarSim2PreScanSTATE/3(z [m]) -> MuxState/3(z [m])
  CarSim2PreScanSTATE/4(dx [m/s]) -> MuxState/4(dx [m/s])
  CarSim2PreScanSTATE/5(dy [m/s]) -> MuxState/5(dy [m/s])
  CarSim2PreScanSTATE/6(dz [m/s]) -> MuxState/6(dz [m/s])
  CarSim2PreScanSTATE/7(R [rad]) -> MuxState/7(R [rad])
  CarSim2PreScanSTATE/8(P [rad]) -> MuxState/8(P [rad])
  CarSim2PreScanSTATE/9(Y [rad]) -> MuxState/9(Y [rad])
  CarSim2PreScan_BUS/1(PreScanBUS_VehicleDynamics) -> State_BUS/1, CarSim2PreScan_ContactAdapter/2(State_Bus)
  CarSim2PreScan_ContactAdapter/1(ContactParams) -> ContactParams/1
  CarSimOut/1 -> Bus Selector/1
  Bus Selector/4 -> Mux/4  "<VehicleCoG_Vx[km/h] (signal 4)>"
  Bus Selector/1 -> Mux/1  "<SprungMass_Pos_Global_x[m] (signal 1)>"
  Bus Selector/2 -> Mux/2  "<SprungMass_Pos_Global_y[m] (signal 2)>"
  Bus Selector/3 -> Mux/3  "<SprungMass_Pos_Global_z[m] (signal 3)>"
  Bus Selector/24 -> Mux/24  "<CarSim_Angle_Wheel_FL_Steer[deg] (signal 24)>"
  Bus Selector/28 -> Mux/28  "<CarSim_Angle_Wheel_RL_Roll[deg] (signal 28)>"
  Bus Selector/11 -> Mux/11  "<CarSim_Pos_Wheel_FL_y[m] (signal 11)>"
  Bus Selector/10 -> Mux/10  "<CarSim_Pos_Wheel_FL_x[m] (signal 10)>"
  Bus Selector/7 -> Mux/7  "<SprungMass_Angle_Global_Roll[deg] (signal 7)>"
  Bus Selector/26 -> Mux/26  "<CarSim_Angle_Wheel_FR_Rot[rev] (signal 26)>"
  Bus Selector/30 -> Mux/30  "<CarSim_Angle_Wheel_RL_Steer[deg] (signal 30)>"
  Bus Selector/31 -> Mux/31  "<CarSim_Angle_Wheel_RR_Roll[deg] (signal 31)>"
  Bus Selector/16 -> Mux/16  "<CarSim_Pos_Wheel_RL_x[m] (signal 16)>"
  Bus Selector/6 -> Mux/6  "<VehicleCoG_Vz[km/h] (signal 6)>"
  Bus Selector/12 -> Mux/12  "<CarSim_Pos_Wheel_FL_z[m] (signal 12)>"
  Bus Selector/21 -> Mux/21  "<CarSim_Pos_Wheel_RR_z[m] (signal 21)>"
  Bus Selector/27 -> Mux/27  "<CarSim_Angle_Wheel_FR_Steer[deg] (signal 27)>"
  Bus Selector/5 -> Mux/5  "<VehicleCoG_Vy[km/h] (signal 5)>"
  Bus Selector/19 -> Mux/19  "<CarSim_Pos_Wheel_RR_x[m] (signal 19)>"
  Bus Selector/23 -> Mux/23  "<CarSim_Angle_Wheel_FL_Rot[rev] (signal 23)>"
  Bus Selector/32 -> Mux/32  "<CarSim_Angle_Wheel_RR_Rot[rev] (signal 32)>"
  Bus Selector/29 -> Mux/29  "<CarSim_Angle_Wheel_RL_Rot[rev] (signal 29)>"
  Bus Selector/35 -> Mux/35  "<Axle1ReducedSW (signal 35)>"
  Bus Selector/13 -> Mux/13  "<CarSim_Pos_Wheel_FR_x[m] (signal 13)>"
  Bus Selector/34 -> Mux/34  "<SteeringWheelAngle[deg] (signal 34)>"
  Bus Selector/9 -> Mux/9  "<SprungMass_Angle_Global_Yaw[deg] (signal 9)>"
  Bus Selector/20 -> Mux/20  "<CarSim_Pos_Wheel_RR_y[m] (signal 20)>"
  Bus Selector/25 -> Mux/25  "<CarSim_Angle_Wheel_FR_Roll[deg] (signal 25)>"
  Bus Selector/8 -> Mux/8  "<SprungMass_Angle_Global_Pitch[deg] (signal 8)>"
  Bus Selector/15 -> Mux/15  "<CarSim_Pos_Wheel_FR_z[m] (signal 15)>"
  Bus Selector/17 -> Mux/17  "<CarSim_Pos_Wheel_RL_y[m] (signal 17)>"
  Bus Selector/18 -> Mux/18  "<CarSim_Pos_Wheel_RL_Z[m] (signal 18)>"
  Bus Selector/14 -> Mux/14  "<CarSim_Pos_Wheel_FR_y[m] (signal 14)>"
  Bus Selector/22 -> Mux/22  "<CarSim_Angle_Wheel_FL_Roll[deg] (signal 22)>"
  Bus Selector/33 -> Mux/33  "<CarSim_Angle_Wheel_RR_Steer[deg] (signal 33)>"
  Mux/1 -> CarSim2PreScan_BUS/1(CarSim_In), Demux/1
  Demux/1 -> CarSim2PreScanSTATE/1(CarSim_In)
  Demux/2 -> Terminator_1/1

== system StraightACC_cs_old/Roewe_550_S_Sedan_1/TIS_1_StandardCoh_Demux ==
  TIS : Inport
  Bus Creator : BusCreator  Inputs=16
  Bus Selector : BusSelector  OutputSignals=ActiveBeamID[-],Range[m],DopplerVelocity[ms-1],DopplerVelocityX[ms-1],DopplerVelocityY[ms-1],DopplerVelocityZ[ms-1],Theta[deg],Phi[deg],TargetID[-],TargetTypeID[-],DopplerVelocityTranslationX[ms-1],DopplerVelocityTranslationY[ms-1],DopplerVelocityTranslationZ[ms-1],DopplerVelocityRotationX[ms-1],DopplerVelocityRotationY[ms-1],DopplerVelocityRotationZ[ms-1]
  ScannerSensorLegacyBusConversion : PreScanUsefulBlocks/ScannerSensorLegacyBusConversion  MAXMESSAGES=MAXMESSAGES
  Out1 : Outport
  Out2 : Outport  Port=2
  Out3 : Outport  Port=3
  Out4 : Outport  Port=4
  Out5 : Outport  Port=5
  Out7 : Outport  Port=6
  Out6 : Outport  Port=7
  wires:
  Bus Selector/16 -> Bus Creator/16  "<DopplerVelocityRotationZ[ms-1]>"
  Bus Selector/15 -> Bus Creator/15  "<DopplerVelocityRotationY[ms-1]>"
  Bus Selector/14 -> Bus Creator/14  "<DopplerVelocityRotationX[ms-1]>"
  Bus Selector/13 -> Bus Creator/13  "<DopplerVelocityTranslationZ[ms-1]>"
  Bus Selector/12 -> Bus Creator/12  "<DopplerVelocityTranslationY[ms-1]>"
  Bus Selector/11 -> Bus Creator/11  "<DopplerVelocityTranslationX[ms-1]>"
  ScannerSensorLegacyBusConversion/1 -> Bus Selector/1
  TIS/1 -> ScannerSensorLegacyBusConversion/1
  Bus Creator/1 -> Out6/1
  Bus Selector/10 -> Bus Creator/10  "<TargetTypeID[-]>"
  Bus Selector/9 -> Out7/1, Bus Creator/9  "<TargetID[-]>"
  Bus Selector/1 -> Out1/1, Bus Creator/1  "<ActiveBeamID[-]>"
  Bus Selector/2 -> Out2/1, Bus Creator/2  "<Range[m]>"
  Bus Selector/7 -> Out4/1, Bus Creator/7  "<Theta[deg]>"
  Bus Selector/8 -> Bus Creator/8, Out5/1  "<Phi[deg]>"
  Bus Selector/3 -> Bus Creator/3, Out3/1  "<DopplerVelocity[ms-1]>"
  Bus Selector/4 -> Bus Creator/4  "<DopplerVelocityX[ms-1]>"
  Bus Selector/5 -> Bus Creator/5  "<DopplerVelocityY[ms-1]>"
  Bus Selector/6 -> Bus Creator/6  "<DopplerVelocityZ[ms-1]>"
